simulink model "PIDmodel"  (R2023b)
settings: Solver=FixedStepAuto  StartTime=0.0  StopTime=200  FixedStep=0.1  RelTol=1e-3
libraries: slpidlib x2, simulink x2, matrix_library x1
settings Model: Creator=Felix_Soong  LastModifiedBy=Felix_Soong

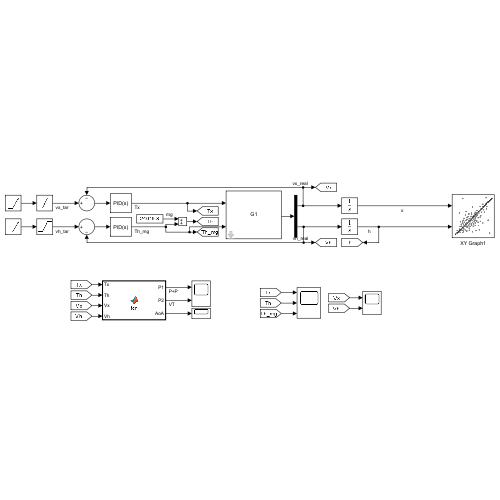
[thumbnail: Simulink's stored preview of the top-level diagram]
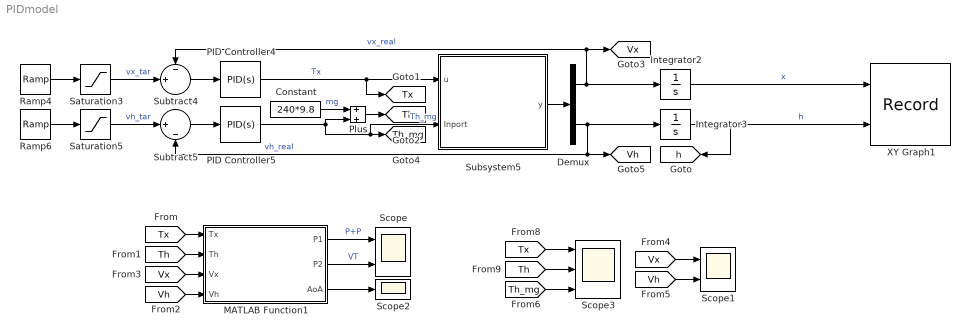
== system PIDmodel ==
  Constant : Constant  Value=240*9.8
  Demux : Demux  Outputs=2
  Integrator2 : Integrator
  Integrator3 : Integrator
  MATLAB Function1 : MATLAB Function  TreatAsAtomicUnit=on
  PID Controller4 : slpidlib/PID Controller  Controller=PID  Form=Parallel  TimeDomain=Continuous-time  UseExternalTs=off  SampleTime=-1  IntegratorMethod=Forward Euler  FilterMethod=Forward Euler  ControllerParametersSource=internal  P=416.552891741816  I=133.885986163438  UseKiTs=off  D=43.4731448254193  N=6.63612888550275  UseFilter=on  TunerSelectOption=Transfer Function Based (PID Tuner App)  InitialConditionSource=internal  InitialConditionForIntegrator=0  InitialConditionForFilter=0  DifferentiatorICPrevScaledInput=0  ExternalReset=none  TrackingMode=off  Kt=1  LimitOutput=off  SatLimitsSource=internal  UpperSaturationLimit=inf  LowerSaturationLimit=-inf  LinearizeAsGain=on  AntiWindupMode=none  Kb=1  LimitIntegrator=off  UpperIntegratorSaturationLimit=inf  LowerIntegratorSaturationLimit=-inf  POutMin=[]  POutMax=[]  IOutMin=[]  IOutMax=[]  DOutMin=[]  DOutMax=[]  NOutMin=[]  NOutMax=[]  SumOutMin=[]  SumOutMax=[]  SaturationOutMin=[]  SaturationOutMax=[]  PParamMin=[]  PParamMax=[]  IParamMin=[]  IParamMax=[]  DParamMin=[]  DParamMax=[]  NParamMin=[]  NParamMax=[]  KbParamMin=[]  KbParamMax=[]  KtParamMin=[]  KtParamMax=[]  KbOutMin=[]  KbOutMax=[]  KtOutMin=[]  KtOutMax=[]  IntegratorOutMin=[]  IntegratorOutMax=[]  FilterOutMin=[]  FilterOutMax=[]  SumI1OutMin=[]  SumI1OutMax=[]  SumI2OutMin=[]  SumI2OutMax=[]  SumI3OutMin=[]  SumI3OutMax=[]  SumI4OutMin=[]  SumI4OutMax=[]  SumDOutMin=[]  SumDOutMax=[]  DifferentiatorOutMin=[]  DifferentiatorOutMax=[]  FilterDiffOutCoefMin=[]  FilterDiffOutCoefMax=[]  ReciprocalOutMin=[]  ReciprocalOutMax=[]  SumDenOutMin=[]  SumDenOutMax=[]  SumNumOutMin=[]  SumNumOutMax=[]  DivideOutMin=[]  DivideOutMax=[]  UdiffTsProdOutMin=[]  UdiffTsProdOutMax=[]  NTsProdOutMin=[]  NTsProdOutMax=[]  UintegralTsProdOutMin=[]  UintegralTsProdOutMax=[]  UngainTsProdOutMin=[]  UngainTsProdOutMax=[]  ClampingZeroOutDataTypeStr=Inherit: Inherit via back propagation  ClampingZeroOutMin=[]  ClampingZeroOutMax=[]  FilterDenConstantOutDataTypeStr=Inherit: Inherit via back propagation  FilterDenConstantOutMin=[]  FilterDenConstantOutMax=[]  PCopyOutDataTypeStr=Inherit: Inherit via back propagation  PCopyOutMin=[]  PCopyOutMax=[]  NCopyOutDataTypeStr=Inherit: Inherit via back propagation  NCopyOutMin=[]  NCopyOutMax=[]  IntegratorContinuousStateAttributes=''  IntegratorStateMustResolveToSignalObject=off  IntegratorRTWStateStorageClass=Auto  FilterContinuousStateAttributes=''  FilterStateMustResolveToSignalObject=off  FilterRTWStateStorageClass=Auto  ParallelPVariant=InternalParameters  IdealPVariant=Disabled  IVariant=InternalParameters  DVariant=InternalParameters  IntegratorVariant=Continuous  SatVariant=Disabled  AWVariant=Passthrough  PCopyVariant=Disabled  TRVariant=Disabled  FdbkBlocksVariant=Forward  IdealPFdbkVariant=Disabled  SatFdbkVariant=Disabled  DerivativeFilterVariant=ContFilter  NVariant=InternalParameters  NCopyVariant=Disabled  FilterICVariant=InternalICsFilter  IntegratorICVariant=InternalICs  ExternalResetVariant=Disabled  TRSumVariant=Passthrough  SumFdbkVariant=Disabled  SumVariant=Sum_PID  TsampFilterVariant=InternalTs  TsampNgainVariant=Passthrough  TsampIntegralVariant=Disabled_SignalSpec  ExternalSaturationOutDataTypeStr=Inherit: Same as second input
  PID Controller5 : slpidlib/PID Controller  Controller=PID  Form=Parallel  TimeDomain=Continuous-time  UseExternalTs=off  SampleTime=-1  IntegratorMethod=Forward Euler  FilterMethod=Forward Euler  ControllerParametersSource=internal  P=1559.8476067563  I=943.53288128348  UseKiTs=off  D=-103.949358808692  N=5.44051767311659  UseFilter=on  TunerSelectOption=Transfer Function Based (PID Tuner App)  InitialConditionSource=internal  InitialConditionForIntegrator=0  InitialConditionForFilter=0  DifferentiatorICPrevScaledInput=0  ExternalReset=none  TrackingMode=off  Kt=1  LimitOutput=off  SatLimitsSource=internal  UpperSaturationLimit=inf  LowerSaturationLimit=-inf  LinearizeAsGain=on  AntiWindupMode=none  Kb=1  LimitIntegrator=off  UpperIntegratorSaturationLimit=inf  LowerIntegratorSaturationLimit=-inf  POutMin=[]  POutMax=[]  IOutMin=[]  IOutMax=[]  DOutMin=[]  DOutMax=[]  NOutMin=[]  NOutMax=[]  SumOutMin=[]  SumOutMax=[]  SaturationOutMin=[]  SaturationOutMax=[]  PParamMin=[]  PParamMax=[]  IParamMin=[]  IParamMax=[]  DParamMin=[]  DParamMax=[]  NParamMin=[]  NParamMax=[]  KbParamMin=[]  KbParamMax=[]  KtParamMin=[]  KtParamMax=[]  KbOutMin=[]  KbOutMax=[]  KtOutMin=[]  KtOutMax=[]  IntegratorOutMin=[]  IntegratorOutMax=[]  FilterOutMin=[]  FilterOutMax=[]  SumI1OutMin=[]  SumI1OutMax=[]  SumI2OutMin=[]  SumI2OutMax=[]  SumI3OutMin=[]  SumI3OutMax=[]  SumI4OutMin=[]  SumI4OutMax=[]  SumDOutMin=[]  SumDOutMax=[]  DifferentiatorOutMin=[]  DifferentiatorOutMax=[]  FilterDiffOutCoefMin=[]  FilterDiffOutCoefMax=[]  ReciprocalOutMin=[]  ReciprocalOutMax=[]  SumDenOutMin=[]  SumDenOutMax=[]  SumNumOutMin=[]  SumNumOutMax=[]  DivideOutMin=[]  DivideOutMax=[]  UdiffTsProdOutMin=[]  UdiffTsProdOutMax=[]  NTsProdOutMin=[]  NTsProdOutMax=[]  UintegralTsProdOutMin=[]  UintegralTsProdOutMax=[]  UngainTsProdOutMin=[]  UngainTsProdOutMax=[]  ClampingZeroOutDataTypeStr=Inherit: Inherit via back propagation  ClampingZeroOutMin=[]  ClampingZeroOutMax=[]  FilterDenConstantOutDataTypeStr=Inherit: Inherit via back propagation  FilterDenConstantOutMin=[]  FilterDenConstantOutMax=[]  PCopyOutDataTypeStr=Inherit: Inherit via back propagation  PCopyOutMin=[]  PCopyOutMax=[]  NCopyOutDataTypeStr=Inherit: Inherit via back propagation  NCopyOutMin=[]  NCopyOutMax=[]  IntegratorContinuousStateAttributes=''  IntegratorStateMustResolveToSignalObject=off  IntegratorRTWStateStorageClass=Auto  FilterContinuousStateAttributes=''  FilterStateMustResolveToSignalObject=off  FilterRTWStateStorageClass=Auto  ParallelPVariant=InternalParameters  IdealPVariant=Disabled  IVariant=InternalParameters  DVariant=InternalParameters  IntegratorVariant=Continuous  SatVariant=Disabled  AWVariant=Passthrough  PCopyVariant=Disabled  TRVariant=Disabled  FdbkBlocksVariant=Forward  IdealPFdbkVariant=Disabled  SatFdbkVariant=Disabled  DerivativeFilterVariant=ContFilter  NVariant=InternalParameters  NCopyVariant=Disabled  FilterICVariant=InternalICsFilter  IntegratorICVariant=InternalICs  ExternalResetVariant=Disabled  TRSumVariant=Passthrough  SumFdbkVariant=Disabled  SumVariant=Sum_PID  TsampFilterVariant=InternalTs  TsampNgainVariant=Passthrough  TsampIntegralVariant=Disabled_SignalSpec  ExternalSaturationOutDataTypeStr=Inherit: Same as second input
  Plus : Sum
  Ramp4 : simulink/Sources/Ramp  slope=0.5  start=50  InitialOutput=0
  Ramp6 : simulink/Sources/Ramp  slope=0.5  start=15  InitialOutput=0
  Saturation3 : Saturate  UpperLimit=50  LowerLimit=0
  Saturation5 : Saturate  UpperLimit=10  LowerLimit=0
  Scope : Scope  NumInputPorts=2
  Scope1 : Scope  NumInputPorts=2
  Scope2 : Scope
  Scope3 : Scope  NumInputPorts=3
  Subsystem5 : Subsystem  mask{m=240, Fx=2.11, Fh=1.47, rou=1.225}
      mask prompts: m "mass"; rou "air density"
      mask DialogControl ParameterGroupVar Prompt: 参数
      mask Display: disp('G1');
  Subtract4 : Sum  Inputs=-|+||
  Subtract5 : Sum  Inputs=||+|-
  XY Graph1 : Record  FileSettingsInternal="{\"entries\":[{\"content\":{\"excelSettings\":{\"content\":{},\"type\":\"Streamout.ExcelSettings\"}},\"type\":\"Streamout.FileSettingStorage\",\"uuid\":\"\"}],\"packageUris\":[\"http:\\/\\/schema.mathworks.com\\/mf0\\/streamout_blocks\\/R2020a\"],\"version\":\"1.0\"}"  Layout=[1 1]  SignalsInternal="{\"entries\":[{\"content\":{\"signals\":[{\"content\":{\"blockPath\":[],\"dimensions\":[1,1],\"domain\":\"\",\"lineColor\":\"#a2142f\",\"plots\":[1],\"port\":1,\"sid\":[\"\"],\"signalID\":2641,\"signalName\":\"x\"},\"type\":\"RecordBlkView.Signal\",\"uuid\":\"\"},{\"content\":{\"blockPath\":[],\"dimensions\":[1,1],\"domain\":\"\",\"lineColor\":\"#139fff\",\"plots\":[1],\"port\":2,\"sid\":[\"\"],\"signalID\":2645,\"signalName\":\"h\"},\"type\":\"RecordBlkView.Signal\",\"uuid\":\"\"}]},\"type\":\"RecordBlkView.InputSignals\",\"uuid\":\"\"}],\"packageUris\":[\"http:\\/\\/schema.mathworks.com\\/mf0\\/streamout_blocks\\/R2020a\"],\"version\":\"1.0\"}"  VisualizationBindings="{\"xyplotplugin\":{\"info\":[{\"series\":[{\"bindingParametersList\":[{\"parameter\":\"X-Axis\",\"signalID\":2641,\"signalName\":\"x\"},{\"parameter\":\"Y-Axis\",\"signalID\":2645,\"signalName\":\"h\"}],\"seriesID\":22818}],\"subplotID\":1}]}}"  CompatibilityTag=XY
  tag scope: Th=global, Th_mg=global, Tx=global, Vh=global, Vx=global, h=global
  wires:
  Saturation5/1 -> Subtract5/1  "vh_tar"
  Subtract5/1 -> PID Controller5/1
  Saturation3/1 -> Subtract4/2  "vx_tar"
  Subtract4/1 -> PID Controller4/1
  Ramp4/1 -> Saturation3/1
  Ramp6/1 -> Saturation5/1
  Subsystem5/1(y) -> Demux/1
  Demux/1 -> Integrator2/1, [Vx], Subtract4/1  "vx_real"
  Demux/2 -> Integrator3/1, [Vh], Subtract5/2  "vh_real"
  Integrator3/1 -> [h], XY Graph1/2  "h"
  Integrator2/1 -> XY Graph1/1  "x"
  PID Controller4/1 -> [Tx], Subsystem5/1(u)  "Tx"
  PID Controller5/1 -> Subsystem5/2(Inport), [Th_mg], Plus/2  "Th_mg"
  [Tx] -> MATLAB Function1/1(Tx)
  [Th] -> MATLAB Function1/2(Th)
  [Vx] -> MATLAB Function1/3(Vx)
  [Vh] -> MATLAB Function1/4(Vh)
  MATLAB Function1/1(P1) -> Scope/1  "P+P"
  MATLAB Function1/2(P2) -> Scope/2  "VT"
  MATLAB Function1/3(AoA) -> Scope2/1
  [Tx] -> Scope3/1
  [Th] -> Scope3/2
  Plus/1 -> [Th]
  Constant/1 -> Plus/1  "mg"
  [Vx] -> Scope1/1
  [Vh] -> Scope1/2
  [Th_mg] -> Scope3/3

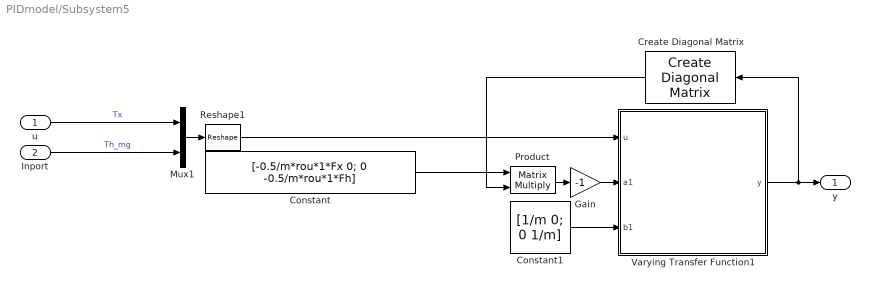
== system PIDmodel/Subsystem5 ==
  u : Inport
  Inport : Inport  Port=2
  Constant : Constant  Value=[-0.5/m*rou*1*Fx 0; 0 -0.5/m*rou*1*Fh]  VectorParams1D=off
  Constant1 : Constant  Value=[1/m 0; 0 1/m]  VectorParams1D=off
  Create Diagonal Matrix : matrix_library/Create Diagonal Matrix
      settings: LibrarySourceBlock=|
      | simulink/Matrix
      | Operations/Create Diagonal
      | Matrix
  Gain : Gain  Gain=-1
  Mux1 : Mux  Inputs=2
  Product : Product  Multiplication=Matrix(*)
  Reshape1 : Reshape  OutputDimensionality=Customize  OutputDimensions=[2,1]
  Varying Transfer Function1 : Subsystem  AncestorBlock=cstblocks/Linear Parameter Varying/Varying Transfer Function  mask(Varying Transfer Function){N=1, Feedthrough=off}
      mask prompts: N "Control:simulink:VaryingTFLabel1"; Feedthrough "Control:simulink:VaryingSSLabel6"
      mask help: Control:simulink:VaryingTF1
      mask init:
      | if N~=round(N)
      |    hCB = get_param(gcb,'handle');
      |    DAStudio.slerror('Control:simulink:InvalidOrder',hCB)
      | end
      | Ts = 0;
      | SimStatus = get_param(bdroot,'SimulationStatus');
      | if any(strcmp(SimStatus,{'initializing','updating','stopped'}))
      |    controllib.internal.blocks.varying.varyingTF(gcb,N,Ts,Feedthrough)
      | end
      mask Help: eval('helpview(''control'',''VaryingTFCT'');')
      mask DialogControl N Prompt: 传递函数阶:
      mask DialogControl Feedthrough Prompt: 启用馈通
      mask Display:
      | port_label('input',2,'a1');
      | port_label('input',3,'b1');
      | plot([0.325 0.675],[0.5 0.5])
      | text(0.5, 0.7, 'b_1 s^{-1}' ,...
      |         'horizontalAlignment', 'center','texmode','on')
      | text(0.5, 0.3, '1 + a_1 s^{-1}' ,...
      |         'horizontalAlignment', 'center','texmode','on')
  y : Outport
  wires:
  Constant1/1 -> Varying Transfer Function1/3(b1)
  Varying Transfer Function1/1(y) -> Create Diagonal Matrix/1, y/1
  Constant/1 -> Product/1
  Create Diagonal Matrix/1 -> Product/2
  Mux1/1 -> Reshape1/1
  u/1 -> Mux1/1  "Tx"
  Reshape1/1 -> Varying Transfer Function1/1(u)
  Inport/1 -> Mux1/2  "Th_mg"
  Product/1 -> Gain/1
  Gain/1 -> Varying Transfer Function1/2(a1)

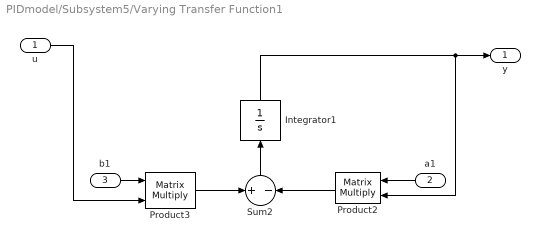
== system PIDmodel/Subsystem5/Varying Transfer Function1 ==
  u : Inport
  a1 : Inport  Port=2
  b1 : Inport  Port=3
  Integrator1 : Integrator
  Product2 : Product  Multiplication=Matrix(*)  InputSameDT=on  RndMeth=Zero  SaturateOnIntegerOverflow=on  OutDataTypeStr=Inherit: Same as first input
  Product3 : Product  Multiplication=Matrix(*)  InputSameDT=on  RndMeth=Zero  SaturateOnIntegerOverflow=on  OutDataTypeStr=Inherit: Same as first input
  Sum2 : Sum  Inputs=+|-  InputSameDT=on  SaturateOnIntegerOverflow=on  OutDataTypeStr=Inherit: Same as first input
  y : Outport  VectorParamsAs1DForOutWhenUnconnected=off
  wires:
  Integrator1/1 -> Product2/2, y/1
  Sum2/1 -> Integrator1/1
  Product3/1 -> Sum2/1
  Product2/1 -> Sum2/2
  b1/1 -> Product3/1
  u/1 -> Product3/2
  a1/1 -> Product2/1

== matlab function PIDmodel/MATLAB Function1 ==
  data: Tx input; P1 output; Th input; Vx input; Vh input; P2 output; AoA output
function [P1, P2, AoA] = fcn(Tx, Th, Vx, Vh)
T = sqrt(Tx^2+Th^2);
V = sqrt(Vx^2+Vh^2);

if Th ~= 0
    theta = atan(Tx/Th);
else
    theta = pi/2;
end

if Vx ~= 0
    gamma = atan(Vh/Vx);
else
    gamma = pi/2;
end

alpha = theta + gamma;
AoA = rad2deg(alpha);

A = 1.6^2 * 3.14;
P1 = T*sqrt(T/(2*1.225*A)) + T*V*sin(alpha);
P2 = T*V;
